simulink library "HWO_lib"  (Simulink 7.5)
settings: Solver=ode45  StartTime=0.0  StopTime=10.0  RelTol=1e-3
libraries: simulink x1
settings Model: Creator=wuaibin  LastModifiedBy=wuaibin

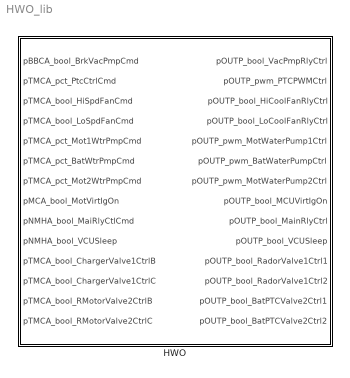
== system HWO_lib ==
  HWO : Subsystem  TreatAsAtomicUnit=on

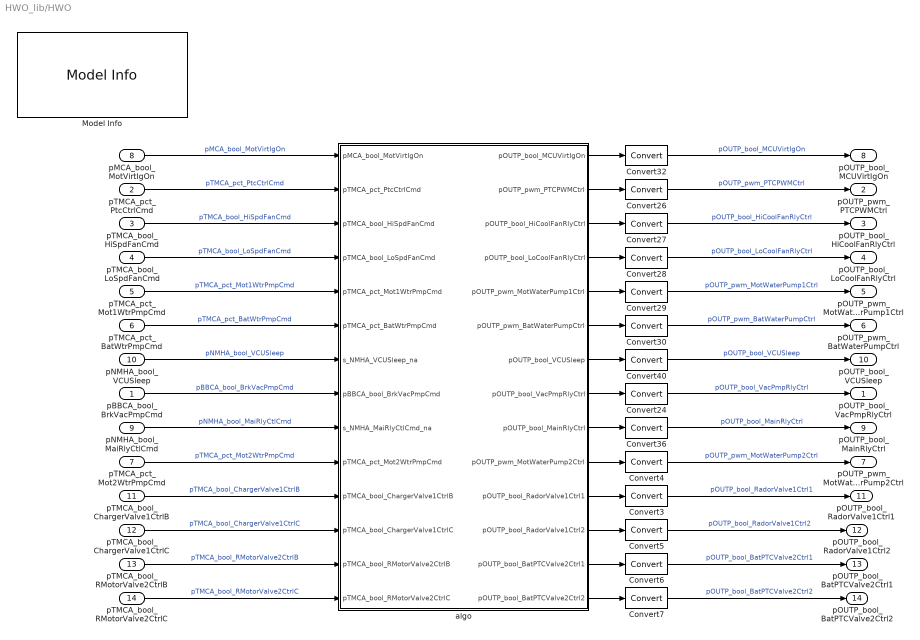
== system HWO_lib/HWO ==
  pBBCA_bool_BrkVacPmpCmd : Inport  OutDataType=fixdt(1, 16)  OutScaling=2^0
  pTMCA_pct_PtcCtrlCmd : Inport  Port=2  OutDataType=fixdt(1, 16)  OutScaling=2^0
  pTMCA_bool_HiSpdFanCmd : Inport  Port=3  OutDataType=fixdt(1, 16)  OutScaling=2^0
  pTMCA_bool_LoSpdFanCmd : Inport  Port=4  OutDataType=fixdt(1, 16)  OutScaling=2^0
  pTMCA_pct_Mot1WtrPmpCmd : Inport  Port=5  OutDataType=fixdt(1, 16)  OutScaling=2^0
  pTMCA_pct_BatWtrPmpCmd : Inport  Port=6  OutDataType=fixdt(1, 16)  OutScaling=2^0
  pTMCA_pct_Mot2WtrPmpCmd : Inport  Port=7  OutDataType=fixdt(1, 16)  OutScaling=2^0
  pMCA_bool_MotVirtIgOn : Inport  Port=8  OutDataType=fixdt(1, 16)  OutScaling=2^0
  pNMHA_bool_MaiRlyCtlCmd : Inport  Port=9  OutDataType=fixdt(1, 16)  OutScaling=2^0
  pNMHA_bool_VCUSleep : Inport  Port=10  OutDataType=fixdt(1, 16)  OutScaling=2^0
  pTMCA_bool_ChargerValve1CtrlB : Inport  Port=11  OutDataType=fixdt(1, 16)  OutScaling=2^0
  pTMCA_bool_ChargerValve1CtrlC : Inport  Port=12  OutDataType=fixdt(1, 16)  OutScaling=2^0
  pTMCA_bool_RMotorValve2CtrlB : Inport  Port=13  OutDataType=fixdt(1, 16)  OutScaling=2^0
  pTMCA_bool_RMotorValve2CtrlC : Inport  Port=14  OutDataType=fixdt(1, 16)  OutScaling=2^0
  Convert{3..7,24,26..30,32,36,40} (14 alike) : DataTypeConversion  OutDataType=fixdt(1, 16)  OutScaling=2^0
  Model Info : simulink/Model-Wide Utilities/Model Info  SystemSampleTime=-1  InitialBlockCM=None  BlockCM=None  Frame=on  DisplayStringWithTags=Model Info\nCreated: %<Created>\nCreator: zhangqiang  HorizontalTextAlignment=Center  LeftAlignmentValue=0.5  SourceBlockDiagram=HQEV_HCU  TagMaxNumber=20
  algo : Subsystem
  pOUTP_bool_VacPmpRlyCtrl : Outport  OutDataType=fixdt(1, 16)  OutScaling=2^0
  pOUTP_pwm_PTCPWMCtrl : Outport  Port=2  OutDataType=fixdt(1, 16)  OutScaling=2^0
  pOUTP_bool_HiCoolFanRlyCtrl : Outport  Port=3  OutDataType=fixdt(1, 16)  OutScaling=2^0
  pOUTP_bool_LoCoolFanRlyCtrl : Outport  Port=4  OutDataType=fixdt(1, 16)  OutScaling=2^0
  pOUTP_pwm_MotWaterPump1Ctrl : Outport  Port=5  OutDataType=fixdt(1, 16)  OutScaling=2^0
  pOUTP_pwm_BatWaterPumpCtrl : Outport  Port=6  OutDataType=fixdt(1, 16)  OutScaling=2^0
  pOUTP_pwm_MotWaterPump2Ctrl : Outport  Port=7  OutDataType=fixdt(1, 16)  OutScaling=2^0
  pOUTP_bool_MCUVirtIgOn : Outport  Port=8  OutDataType=fixdt(1, 16)  OutScaling=2^0
  pOUTP_bool_MainRlyCtrl : Outport  Port=9  OutDataType=fixdt(1, 16)  OutScaling=2^0
  pOUTP_bool_VCUSleep : Outport  Port=10  OutDataType=fixdt(1, 16)  OutScaling=2^0
  pOUTP_bool_RadorValve1Ctrl1 : Outport  Port=11
  pOUTP_bool_RadorValve1Ctrl2 : Outport  Port=12
  pOUTP_bool_BatPTCValve2Ctrl1 : Outport  Port=13
  pOUTP_bool_BatPTCValve2Ctrl2 : Outport  Port=14
  wires:
  pTMCA_bool_RMotorValve2CtrlC/1 -> algo/14(pTMCA_bool_RMotorValve2CtrlC)  "pTMCA_bool_RMotorValve2CtrlC"
  pTMCA_bool_RMotorValve2CtrlB/1 -> algo/13(pTMCA_bool_RMotorValve2CtrlB)  "pTMCA_bool_RMotorValve2CtrlB"
  pTMCA_bool_ChargerValve1CtrlC/1 -> algo/12(pTMCA_bool_ChargerValve1CtrlC)  "pTMCA_bool_ChargerValve1CtrlC"
  pTMCA_bool_ChargerValve1CtrlB/1 -> algo/11(pTMCA_bool_ChargerValve1CtrlB)  "pTMCA_bool_ChargerValve1CtrlB"
  Convert7/1 -> pOUTP_bool_BatPTCValve2Ctrl2/1  "pOUTP_bool_BatPTCValve2Ctrl2"
  Convert6/1 -> pOUTP_bool_BatPTCValve2Ctrl1/1  "pOUTP_bool_BatPTCValve2Ctrl1"
  Convert5/1 -> pOUTP_bool_RadorValve1Ctrl2/1  "pOUTP_bool_RadorValve1Ctrl2"
  Convert3/1 -> pOUTP_bool_RadorValve1Ctrl1/1  "pOUTP_bool_RadorValve1Ctrl1"
  algo/14(pOUTP_bool_BatPTCValve2Ctrl2) -> Convert7/1
  algo/13(pOUTP_bool_BatPTCValve2Ctrl1) -> Convert6/1
  algo/12(pOUTP_bool_RadorValve1Ctrl2) -> Convert5/1
  algo/11(pOUTP_bool_RadorValve1Ctrl1) -> Convert3/1
  algo/10(pOUTP_pwm_MotWaterPump2Ctrl) -> Convert4/1
  pTMCA_pct_Mot2WtrPmpCmd/1 -> algo/10(pTMCA_pct_Mot2WtrPmpCmd)  "pTMCA_pct_Mot2WtrPmpCmd"
  Convert4/1 -> pOUTP_pwm_MotWaterPump2Ctrl/1  "pOUTP_pwm_MotWaterPump2Ctrl"
  Convert40/1 -> pOUTP_bool_VCUSleep/1  "pOUTP_bool_VCUSleep"
  pNMHA_bool_VCUSleep/1 -> algo/7(s_NMHA_VCUSleep_na)  "pNMHA_bool_VCUSleep"
  algo/7(pOUTP_bool_VCUSleep) -> Convert40/1
  algo/8(pOUTP_bool_VacPmpRlyCtrl) -> Convert24/1
  Convert24/1 -> pOUTP_bool_VacPmpRlyCtrl/1  "pOUTP_bool_VacPmpRlyCtrl"
  pBBCA_bool_BrkVacPmpCmd/1 -> algo/8(pBBCA_bool_BrkVacPmpCmd)  "pBBCA_bool_BrkVacPmpCmd"
  algo/2(pOUTP_pwm_PTCPWMCtrl) -> Convert26/1
  Convert26/1 -> pOUTP_pwm_PTCPWMCtrl/1  "pOUTP_pwm_PTCPWMCtrl"
  pTMCA_pct_PtcCtrlCmd/1 -> algo/2(pTMCA_pct_PtcCtrlCmd)  "pTMCA_pct_PtcCtrlCmd"
  algo/3(pOUTP_bool_HiCoolFanRlyCtrl) -> Convert27/1
  Convert27/1 -> pOUTP_bool_HiCoolFanRlyCtrl/1  "pOUTP_bool_HiCoolFanRlyCtrl"
  pTMCA_bool_HiSpdFanCmd/1 -> algo/3(pTMCA_bool_HiSpdFanCmd)  "pTMCA_bool_HiSpdFanCmd"
  algo/4(pOUTP_bool_LoCoolFanRlyCtrl) -> Convert28/1
  Convert28/1 -> pOUTP_bool_LoCoolFanRlyCtrl/1  "pOUTP_bool_LoCoolFanRlyCtrl"
  pTMCA_bool_LoSpdFanCmd/1 -> algo/4(pTMCA_bool_LoSpdFanCmd)  "pTMCA_bool_LoSpdFanCmd"
  algo/5(pOUTP_pwm_MotWaterPump1Ctrl) -> Convert29/1
  Convert29/1 -> pOUTP_pwm_MotWaterPump1Ctrl/1  "pOUTP_pwm_MotWaterPump1Ctrl"
  pTMCA_pct_Mot1WtrPmpCmd/1 -> algo/5(pTMCA_pct_Mot1WtrPmpCmd)  "pTMCA_pct_Mot1WtrPmpCmd"
  algo/6(pOUTP_pwm_BatWaterPumpCtrl) -> Convert30/1
  Convert30/1 -> pOUTP_pwm_BatWaterPumpCtrl/1  "pOUTP_pwm_BatWaterPumpCtrl"
  pTMCA_pct_BatWtrPmpCmd/1 -> algo/6(pTMCA_pct_BatWtrPmpCmd)  "pTMCA_pct_BatWtrPmpCmd"
  algo/1(pOUTP_bool_MCUVirtIgOn) -> Convert32/1
  Convert32/1 -> pOUTP_bool_MCUVirtIgOn/1  "pOUTP_bool_MCUVirtIgOn"
  pMCA_bool_MotVirtIgOn/1 -> algo/1(pMCA_bool_MotVirtIgOn)  "pMCA_bool_MotVirtIgOn"
  algo/9(pOUTP_bool_MainRlyCtrl) -> Convert36/1
  Convert36/1 -> pOUTP_bool_MainRlyCtrl/1  "pOUTP_bool_MainRlyCtrl"
  pNMHA_bool_MaiRlyCtlCmd/1 -> algo/9(s_NMHA_MaiRlyCtlCmd_na)  "pNMHA_bool_MaiRlyCtlCmd"

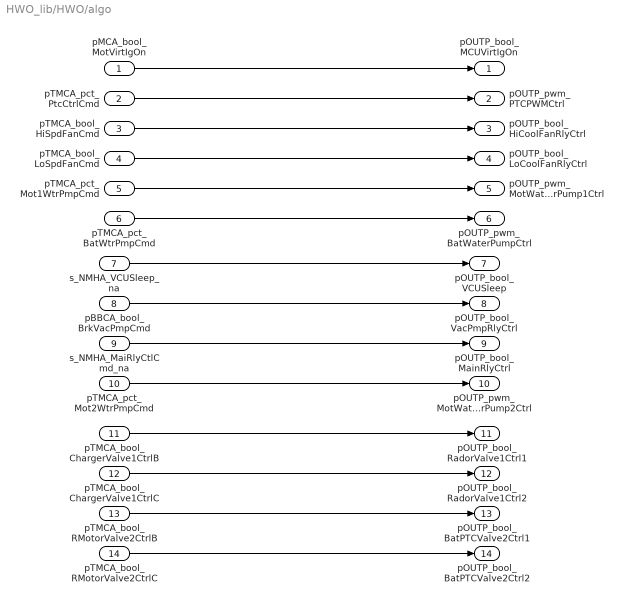
== system HWO_lib/HWO/algo ==
  pMCA_bool_MotVirtIgOn : Inport  OutDataType=fixdt(1, 16)  OutScaling=2^0
  pTMCA_pct_PtcCtrlCmd : Inport  Port=2  OutDataType=fixdt(1, 16)  OutScaling=2^0
  pTMCA_bool_HiSpdFanCmd : Inport  Port=3  OutDataType=fixdt(1, 16)  OutScaling=2^0
  pTMCA_bool_LoSpdFanCmd : Inport  Port=4  OutDataType=fixdt(1, 16)  OutScaling=2^0
  pTMCA_pct_Mot1WtrPmpCmd : Inport  Port=5  OutDataType=fixdt(1, 16)  OutScaling=2^0
  pTMCA_pct_BatWtrPmpCmd : Inport  Port=6  OutDataType=fixdt(1, 16)  OutScaling=2^0
  s_NMHA_VCUSleep_na : Inport  Port=7  OutDataType=fixdt(1, 16)  OutScaling=2^0
  pBBCA_bool_BrkVacPmpCmd : Inport  Port=8  OutDataType=fixdt(1, 16)  OutScaling=2^0
  s_NMHA_MaiRlyCtlCmd_na : Inport  Port=9  OutDataType=fixdt(1, 16)  OutScaling=2^0
  pTMCA_pct_Mot2WtrPmpCmd : Inport  Port=10  OutDataType=fixdt(1, 16)  OutScaling=2^0
  pTMCA_bool_ChargerValve1CtrlB : Inport  Port=11  OutDataType=fixdt(1, 16)  OutScaling=2^0
  pTMCA_bool_ChargerValve1CtrlC : Inport  Port=12  OutDataType=fixdt(1, 16)  OutScaling=2^0
  pTMCA_bool_RMotorValve2CtrlB : Inport  Port=13  OutDataType=fixdt(1, 16)  OutScaling=2^0
  pTMCA_bool_RMotorValve2CtrlC : Inport  Port=14  OutDataType=fixdt(1, 16)  OutScaling=2^0
  pOUTP_bool_MCUVirtIgOn : Outport  OutDataType=fixdt(1, 16)  OutScaling=2^0
  pOUTP_pwm_PTCPWMCtrl : Outport  Port=2  OutDataType=fixdt(1, 16)  OutScaling=2^0
  pOUTP_bool_HiCoolFanRlyCtrl : Outport  Port=3  OutDataType=fixdt(1, 16)  OutScaling=2^0
  pOUTP_bool_LoCoolFanRlyCtrl : Outport  Port=4  OutDataType=fixdt(1, 16)  OutScaling=2^0
  pOUTP_pwm_MotWaterPump1Ctrl : Outport  Port=5  OutDataType=fixdt(1, 16)  OutScaling=2^0
  pOUTP_pwm_BatWaterPumpCtrl : Outport  Port=6  OutDataType=fixdt(1, 16)  OutScaling=2^0
  pOUTP_bool_VCUSleep : Outport  Port=7  OutDataType=fixdt(1, 16)  OutScaling=2^0
  pOUTP_bool_VacPmpRlyCtrl : Outport  Port=8  OutDataType=fixdt(1, 16)  OutScaling=2^0
  pOUTP_bool_MainRlyCtrl : Outport  Port=9  OutDataType=fixdt(1, 16)  OutScaling=2^0
  pOUTP_pwm_MotWaterPump2Ctrl : Outport  Port=10  OutDataType=fixdt(1, 16)  OutScaling=2^0
  pOUTP_bool_RadorValve1Ctrl1 : Outport  Port=11
  pOUTP_bool_RadorValve1Ctrl2 : Outport  Port=12
  pOUTP_bool_BatPTCValve2Ctrl1 : Outport  Port=13
  pOUTP_bool_BatPTCValve2Ctrl2 : Outport  Port=14
  wires:
  pTMCA_bool_ChargerValve1CtrlC/1 -> pOUTP_bool_RadorValve1Ctrl2/1
  pTMCA_bool_ChargerValve1CtrlB/1 -> pOUTP_bool_RadorValve1Ctrl1/1
  pTMCA_bool_RMotorValve2CtrlB/1 -> pOUTP_bool_BatPTCValve2Ctrl1/1
  pTMCA_bool_RMotorValve2CtrlC/1 -> pOUTP_bool_BatPTCValve2Ctrl2/1
  pTMCA_pct_Mot2WtrPmpCmd/1 -> pOUTP_pwm_MotWaterPump2Ctrl/1
  s_NMHA_MaiRlyCtlCmd_na/1 -> pOUTP_bool_MainRlyCtrl/1
  pBBCA_bool_BrkVacPmpCmd/1 -> pOUTP_bool_VacPmpRlyCtrl/1
  s_NMHA_VCUSleep_na/1 -> pOUTP_bool_VCUSleep/1
  pTMCA_pct_BatWtrPmpCmd/1 -> pOUTP_pwm_BatWaterPumpCtrl/1
  pTMCA_pct_Mot1WtrPmpCmd/1 -> pOUTP_pwm_MotWaterPump1Ctrl/1
  pTMCA_bool_LoSpdFanCmd/1 -> pOUTP_bool_LoCoolFanRlyCtrl/1
  pTMCA_bool_HiSpdFanCmd/1 -> pOUTP_bool_HiCoolFanRlyCtrl/1
  pTMCA_pct_PtcCtrlCmd/1 -> pOUTP_pwm_PTCPWMCtrl/1
  pMCA_bool_MotVirtIgOn/1 -> pOUTP_bool_MCUVirtIgOn/1
